simulink model "suspensao"  (R2015a)
settings: Solver=ode23t  StartTime=0.0  StopTime=10.0  RelTol=1e-3
settings Model: Creator=Joacy Mesquita  LastModifiedBy=Joacy Mesquita

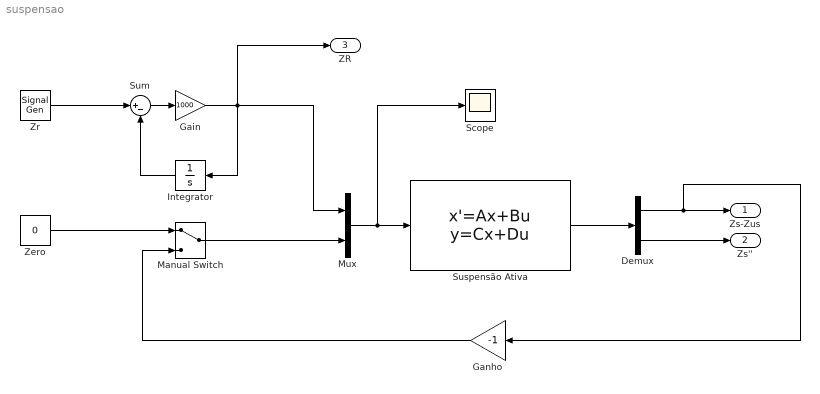
== system suspensao ==
  Demux : Demux  Outputs=2
  Gain : Gain  Gain=1000
  Ganho : Gain  Gain=-1
  Integrator : Integrator
  Manual Switch : ManualSwitch
  Mux : Mux  Inputs=2
  Scope : Scope
  Sum : Sum  Inputs=|+-
  Suspensão Ativa : StateSpace  A=[0 1 0 -1;-367.346938775510 -3.06122448979592 0 3.06122448979592;0 0 0 1;900 7.50000000000000 -1250 -12.5000000000000]  B=[0 0;0 0.408163265306122;-1 0;5 -1]  C=[1 0 0 0;-367.346938775510 -3.06122448979592 0 3.06122448979592]  D=[0 0;0 0.408163265306122]  X0=0
  Zero : Constant  Value=0
  Zr : SignalGenerator  WaveForm=square  Amplitude=-0.01  Frequency=0.3
  Zs-Zus : Outport
  Zs'' : Outport  Port=2
  ZR : Outport  Port=3
  wires:
  Suspensão Ativa/1 -> Demux/1
  Demux/2 -> Zs''/1
  Zr/1 -> Sum/1
  Zero/1 -> Manual Switch/1
  Manual Switch/1 -> Mux/2
  Ganho/1 -> Manual Switch/2
  Gain/1 -> ZR/1, Integrator/1, Mux/1
  Sum/1 -> Gain/1
  Integrator/1 -> Sum/2
  Demux/1 -> Ganho/1, Zs-Zus/1
  Mux/1 -> Scope/1, Suspensão Ativa/1
